simulink model "controlMCUSlugsMKII"  (Simulink 6.6)
settings: Solver=FixedStepDiscrete  StartTime=0.0  StopTime=10.0  FixedStep=0.01  RelTol=1e-3
InitFcn:
  | mcuInit
values from neighbouring files (symbols this model uses):
  apSampleTime = 0.01    [mcuInit.m]
  derivativesConstant = 5    [mcuInit.m]
  T = 0.01    [mcuInit.m]
undefined symbols (not defined in the file or in its folder): bankCommandLimit, baseHeight, bda, bde, bdr, bdt, bICda, bICde, bICdr, bICdt, controlMCUInit, daLimit, deLimit, drLimit, dtLimit, getAccBias, getAccels, getAttitude, getMidLevelCommands, getPassValues, getPidIdx, getVned, getWP, getXYZ, gsRead, ISA_g, lowRateTelemetryMavlink, mda, mde, mdr, mdt, mICda, mICde, mICdr, mICdt, pitchCommandLimit, protDecodeMavlink, readIpc, send2GS, setCurrentCommands, setDiagnosticFloat, setDiagnosticShort, setLogFloat1, setLogFloat2, setNavLat, setNavLong, setNavNav, u1, u2, updateEuler, updateLoad, updatePQR, updatePWM, updatePWM2, y1
libraries: dsPICdrivers x85, simulink x79, SLUGS_Library x23, aerolibconvert2 x5, aerolibutil x3
(part 4 of 5)

== system controlMCUSlugsMKII/Inner Loop/ Navigation/Lateral Channel/Bank to Psi Dot/Protect NaNs1 ==
  In1 : Inport
  Integer Delay3 : simulink/Discrete/Integer Delay  Orientation=left  vinit=0.0  samptime=T  NumDelays=1
  Relational Operator2 : RelationalOperator  Operator===  LogicOutDataTypeMode=Specify via dialog
  Switch3 : Switch  Criteria=u2 > Threshold  Threshold=0.3  SampleTime=.01
  Out1 : Outport  Orientation=down
  wires:
  Integer Delay3/1 -> Switch3/3
  Switch3/1 -> Out1/1, Integer Delay3/1
  In1/1 -> Relational Operator2/2, Relational Operator2/1, Switch3/1
  Relational Operator2/1 -> Switch3/2

== system controlMCUSlugsMKII/Inner Loop/ Navigation/Lateral Channel/Sideslip Compensation/Bank to Psi Dot ==
  phi_c : Inport
  U_m : Inport  Port=2
  Constant1 : Constant  Value=9.80665  OutDataTypeMode=single
  Divide : Product  Inputs=/*  OutDataTypeMode=single  OutScaling=2^-10  SampleTime=apSampleTime
  Divide1 : Product  OutDataTypeMode=single  OutScaling=2^-10  SampleTime=apSampleTime
  Subsystem8 : SLUGS_Library/Subsystem8  SystemSampleTime=-1
  bank Limit : Saturate  UpperLimit=bankCommandLimit  LowerLimit=-bankCommandLimit
  negprotect : Stateflow chart
  psi_dot_c : Outport
  wires:
  U_m/1 -> negprotect/1(val)
  Constant1/1 -> Divide/2
  Divide1/1 -> psi_dot_c/1
  Subsystem8/1 -> Divide1/1
  phi_c/1 -> bank Limit/1
  Divide/1 -> Divide1/2
  negprotect/1(zpVal) -> Divide/1
  bank Limit/1 -> Subsystem8/1

== system controlMCUSlugsMKII/Inner Loop/ Navigation/Lateral Channel/Sideslip Compensation/Low Pass ==
  a : Inport
  u : Inport  Port=2
  Compute Coef : Subsystem
  Detect Change : Subsystem
  Divide : Product  OutScaling=2^-10  SampleTime=apSampleTime
  Divide1 : Product  OutScaling=2^-10  SampleTime=apSampleTime
  IC : InitialCondition
  Integer Delay : simulink/Discrete/Integer Delay  vinit=0.0  samptime=apSampleTime  NumDelays=1
  Integer Delay1 : simulink/Discrete/Integer Delay  Orientation=left  vinit=0.0  samptime=apSampleTime  NumDelays=1
  Subtract : Sum  OutScaling=2^-10  SampleTime=apSampleTime
  y : Outport
  wires:
  Integer Delay1/1 -> Divide1/2
  u/1 -> Integer Delay/1
  IC/1 -> Compute Coef/Enable
  Subtract/1 -> Integer Delay1/1, y/1
  Divide1/1 -> Subtract/2
  Divide/1 -> Subtract/1
  Integer Delay/1 -> Divide/2
  Detect Change/1(change?) -> IC/1
  Compute Coef/2(c) -> Divide1/1
  Compute Coef/1(b) -> Divide/1
  a/1 -> Detect Change/1(Data), Compute Coef/1(a)

== system controlMCUSlugsMKII/Inner Loop/ Navigation/Lateral Channel/Sideslip Compensation/Protect NaNs2 ==
  In1 : Inport
  Integer Delay3 : simulink/Discrete/Integer Delay  Orientation=left  vinit=0.0  samptime=T  NumDelays=1
  Relational Operator2 : RelationalOperator  Operator===  LogicOutDataTypeMode=Specify via dialog
  Switch3 : Switch  Criteria=u2 > Threshold  Threshold=0.3  SampleTime=.01
  Out1 : Outport  Orientation=down
  wires:
  Relational Operator2/1 -> Switch3/2
  In1/1 -> Switch3/1, Relational Operator2/1, Relational Operator2/2
  Switch3/1 -> Integer Delay3/1, Out1/1
  Integer Delay3/1 -> Switch3/3

== system controlMCUSlugsMKII/Inner Loop/ Navigation/Lateral Channel/Sideslip Compensation/psi_dot to Bank ==
  psi_dot_c : Inport
  U_m : Inport  Port=2
  Constant1 : Constant  Value=9.80665  OutDataTypeMode=single
  Divide : Product  Inputs=**/  OutScaling=2^-10  SampleTime=apSampleTime
  Subsystem2 : SLUGS_Library/Subsystem2  SystemSampleTime=-1
  phi_c : Outport
  wires:
  psi_dot_c/1 -> Divide/1
  U_m/1 -> Divide/2
  Constant1/1 -> Divide/3
  Subsystem2/1 -> phi_c/1
  Divide/1 -> Subsystem2/1

== system controlMCUSlugsMKII/Inner Loop/ Navigation/Longitudinal Channel/Air Density from Height/Subsystem ==
  u : Inport
  v : Inport  Port=2
  C Function Call : dsPICdrivers/OTHERS/C Function Call  Tag=dsPIC_dsPIC_CFunctionCall  fctName='myPow'  INPUT_SIZE=1  INPUT1=real32  INPUT2=real32  INPUT3=--  OUTPUT_SIZE=1  OUTPUT1=real32  SampleTime=-1  InputType=[ 7 7 ]  OutputType=[ 7 ]  FctDeclaration=extern real32_T myPow(real32_T u1, real32_T u2);  FctCall=%y1 = myPow(%u1, %u2);  OrderingInOutPopup=None
  u^v : Outport
  wires:
  v/1 -> C Function Call/2
  u/1 -> C Function Call/1
  C Function Call/1 -> u^v/1

== system controlMCUSlugsMKII/Inner Loop/ Navigation/Longitudinal Channel/Airspeed Hold [PID]/Trapezoidal Integrator ==
  x : Inport
  Reset : Inport  Port=2
  Constant : Constant  Value=1/3  OutDataTypeMode=single
  Constant1 : Constant  Value=4/3  OutDataTypeMode=single
  Constant2 : Constant  Value=T/2  OutDataTypeMode=single
  Constant3 : Constant  Value=1/3  OutDataTypeMode=single
  Constant5 : Constant  Orientation=left  Value=0  OutDataTypeMode=single
  Integer Delay : simulink/Discrete/Integer Delay  vinit=0.0  samptime=T  NumDelays=1
  Integer Delay1 : simulink/Discrete/Integer Delay  vinit=0.0  samptime=T  NumDelays=2
  Integer Delay2 : simulink/Discrete/Integer Delay  Orientation=left  vinit=0.0  samptime=T  NumDelays=1
  Product{,1..3} (4 alike) : Product  OutDataTypeMode=single  RndMeth=Zero
  "Protect NaNs " : Subsystem
  Protect NaNs1 : Subsystem
  Subtract : Sum  Inputs=3  OutDataTypeMode=single  OutScaling=2^-10
  Subtract1 : Sum  Inputs=2  OutDataTypeMode=single  OutScaling=2^-10
  Switch1 : Switch  Criteria=u2 > Threshold  Threshold=0.3  SampleTime=.01
  Int(x) : Outport
  wires:
  "Protect NaNs "/1(Out1) -> Product/1, Integer Delay/1, Integer Delay1/1
  Protect NaNs1/1(Out1) -> Int(x)/1, Integer Delay2/1
  Constant/1 -> Product/2
  Constant1/1 -> Product1/2
  Integer Delay/1 -> Product1/1
  Integer Delay1/1 -> Product2/1
  Constant3/1 -> Product2/2
  x/1 -> "Protect NaNs "/1(In1)
  Product/1 -> Subtract/1
  Product1/1 -> Subtract/2
  Product2/1 -> Subtract/3
  Constant2/1 -> Product3/1
  Subtract/1 -> Product3/2
  Subtract1/1 -> Switch1/3
  Integer Delay2/1 -> Subtract1/1
  Product3/1 -> Subtract1/2
  Constant5/1 -> Switch1/1
  Reset/1 -> Switch1/2
  Switch1/1 -> Protect NaNs1/1(In1)

== system controlMCUSlugsMKII/Inner Loop/ Navigation/Longitudinal Channel/Compute Airspeed/Subsystem1 ==
  x : Inport
  C Function Call : dsPICdrivers/OTHERS/C Function Call  Tag=dsPIC_dsPIC_CFunctionCall  fctName='mySqrt'  INPUT_SIZE=1  INPUT1=real32  INPUT2=--  INPUT3=--  OUTPUT_SIZE=1  OUTPUT1=real32  SampleTime=-1  InputType=[ 7 ]  OutputType=[ 7 ]  FctDeclaration=extern real32_T mySqrt(real32_T u1);  FctCall=%y1 = mySqrt(%u1);  OrderingInOutPopup=None
  negprotect : Stateflow chart
  sqrt(x) : Outport
  wires:
  x/1 -> negprotect/1(val)
  negprotect/1(zpVal) -> C Function Call/1
  C Function Call/1 -> sqrt(x)/1

== system controlMCUSlugsMKII/Inner Loop/ Navigation/Navigation/Compute Lateral Error/Subsystem3 ==
  x : Inport
  y : Inport  Port=2
  Dot Product : simulink/Math Operations/Dot Product  InputSameDT=on  OutDataType=sfix(16)  OutScaling=2^-10  DoSatur=off
  Embedded MATLAB Function : Stateflow chart
  Environment Controller : simulink/Signal Routing/Environment Controller  SystemSampleTime=-1
  Protect NaNs : Subsystem
  x dot y : Outport
  wires:
  Environment Controller/1 -> Protect NaNs/1(In1)
  Embedded MATLAB Function/1(xDoty) -> Environment Controller/2
  Dot Product/1 -> Environment Controller/1
  x/1 -> Dot Product/1, Embedded MATLAB Function/1(x)
  y/1 -> Dot Product/2, Embedded MATLAB Function/2(y)
  Protect NaNs/1(Out1) -> x dot y/1

== system controlMCUSlugsMKII/Inner Loop/ Navigation/Navigation/Compute WP Index/Compute P ==
  WP1 : Inport  Orientation=left
  T1 : Inport  Port=2
  WP2 : Inport  Orientation=left  Port=3
  U_com : Inport  Port=4
  GS R_in : Inport  Orientation=left  Port=5
  GS LLA : Inport  Orientation=left  Port=6
  Groundspeed : Inport  Port=7
  Preturn Constant : Inport  Port=8
  Enable : EnablePort
  Add : Sum  Inputs=2  OutScaling=2^-10
  Compute R : Subsystem
  Compute T  in Frenet : Subsystem  Orientation=left  AncestorBlock=SLUGS_Library/Navigation/Compute Frenet
  Demux : Demux  Orientation=left  Outputs=3
  Geod2LTP1 : Subsystem  Orientation=left
      mask Description:
      | This block provides transformation of the Geodetic coordinates
      | to the LTP coorinate system. The block uses two consecutive transformations
      | (Geodetic -> ECEF ->LTP).
      | Geodetic coordinates of the LTP origin should also be predetermined.
      mask Help: Oops!
      mask Display: plot(0,0,100,100,[45,40,35,40,40],[85,95,85,95,40],[85,95,85,95,40],[35,40,45,40,40],[60,40,10,20,10,14],[70,40,10,13,10,20],[56,45],[70,70],[60,60],[50,60],[60,60],[30,40],[50,60],[20,20],[30,40],[20,20],[45,55],[35,25],[75,65],[35,25])
  Get Circles : Subsystem
  IC : InitialCondition  Value=50
  Integer Delay1 : simulink/Discrete/Integer Delay  vinit=0.0  samptime=-1  NumDelays=1
  Integer Delay2 : simulink/Discrete/Integer Delay  Orientation=left  vinit=0.0  samptime=-1  NumDelays=1
  Product1 : Product  OutDataTypeMode=single  RndMeth=Zero
  WP1_1 : InportShadow  Port=1  LatchByCopyingInsideSignal=off
  get WP Coord from Index : Subsystem  Orientation=left  AncestorBlock=SLUGS_Library/Navigation/get WP Coord from Index
  P : Outport  InitialOutput=50
  wires:
  IC/1 -> P/1
  GS LLA/1 -> Geod2LTP1/1(GS Lat,Lon)
  GS R_in/1 -> Geod2LTP1/2(GS ECEF)
  get WP Coord from Index/1(WP Coord) -> Demux/1
  Geod2LTP1/1("NEU, m") -> Integer Delay2/1
  Demux/3 -> Geod2LTP1/5(Hight,m(GPS))
  Demux/2 -> Geod2LTP1/4("Lon, deg(GPS)")
  Demux/1 -> Geod2LTP1/3("Lat, deg(GPS)")
  Integer Delay1/1 -> Get Circles/1(T1)
  WP1_1/1 -> Get Circles/3("Wp_to ")
  T1/1 -> Integer Delay1/1
  WP2/1 -> get WP Coord from Index/1(WP Idx)
  WP1/1 -> Compute T  in Frenet/1(Pos 1)
  Compute T  in Frenet/1(T) -> Get Circles/2(T2)
  Integer Delay2/1 -> Compute T  in Frenet/2(Pos 2)
  Compute R/1(R) -> Get Circles/4(R)
  U_com/1 -> Compute R/1(U_com)
  Product1/1 -> Add/1
  Groundspeed/1 -> Product1/2
  Preturn Constant/1 -> Product1/1
  Get Circles/1(P) -> Add/2
  Add/1 -> IC/1

== system controlMCUSlugsMKII/Inner Loop/ Navigation/Navigation/Compute WP Index/Grab IC ==
  UAV Pos : Inport
  Enable : EnablePort
  Compute GS Location : Subsystem
  Constant : Constant  Value=11  OutDataTypeMode=uint8
  Selector : Selector  IndexOptions=Index vector (dialog)  Indices=[3 1 2]  OutputSizes=1  InputPortWidth=3
  get GS Location (WP 11 is GS) : Subsystem  AncestorBlock=SLUGS_Library/Navigation/get WP Coord from Index
  IC : Outport
  "GS, Lat Lon" : Outport  Port=2
  GS R_in : Outport  Port=3
  wires:
  get GS Location (WP 11 is GS)/1(WP Coord) -> Selector/1
  Selector/1 -> Compute GS Location/1(GS Location)
  Compute GS Location/2(R_in) -> GS R_in/1
  Compute GS Location/1("Lat, Lon") -> "GS, Lat Lon"/1
  Constant/1 -> get GS Location (WP 11 is GS)/1(WP Idx)
  UAV Pos/1 -> IC/1

== system controlMCUSlugsMKII/Inner Loop/ Navigation/Navigation/Compute WP Index/Protect NaNs ==
  In1 : Inport
  Integer Delay3 : simulink/Discrete/Integer Delay  Orientation=left  vinit=0.0  samptime=T  NumDelays=1
  Relational Operator2 : RelationalOperator  Operator===  LogicOutDataTypeMode=Specify via dialog
  Switch3 : Switch  Criteria=u2 > Threshold  Threshold=0.3  SampleTime=.01
  Out1 : Outport  Orientation=down
  wires:
  Relational Operator2/1 -> Switch3/2
  In1/1 -> Switch3/1, Relational Operator2/1, Relational Operator2/2
  Switch3/1 -> Integer Delay3/1, Out1/1
  Integer Delay3/1 -> Switch3/3

== system controlMCUSlugsMKII/Inner Loop/ Navigation/Navigation/Compute WP Index/Subsystem ==
  WP Fly : Inport
  Add1 : Sum  Inputs=2  OutScaling=2^-10
  Hit  Crossing1 : HitCross  HitCrossingOffset=0.3  HitCrossingDirection=rising  SampleTime=apSampleTime
  Integer Delay1 : simulink/Discrete/Integer Delay  vinit=0  samptime=-1  NumDelays=1
  Just Enab : Outport
  wires:
  WP Fly/1 -> Hit  Crossing1/1
  Add1/1 -> Just Enab/1
  Hit  Crossing1/1 -> Integer Delay1/1, Add1/2
  Integer Delay1/1 -> Add1/1

== system controlMCUSlugsMKII/Inner Loop/ Navigation/Navigation/Compute WP Index/Subsystem1 ==
  swInc : Inport  Orientation=down
  Add : Sum  Orientation=left  Inputs=2  OutScaling=2^-10
  IC : InitialCondition  Orientation=down
  Integer Delay2 : simulink/Discrete/Integer Delay  Orientation=left  vinit=0  samptime=-1  NumDelays=1
  swEna : Outport  Orientation=left
  wires:
  swInc/1 -> IC/1
  Add/1 -> swEna/1
  IC/1 -> Add/2, Integer Delay2/1
  Integer Delay2/1 -> Add/1

== system controlMCUSlugsMKII/Inner Loop/ Navigation/Navigation/Compute WP Index/Switch when  in Line Segment ==
  P : Inport
  WP0 Idx : Inport  Port=2
  Puav : Inport  Port=3
  "WP1 " : Inport  Port=4
  WP0 : Inport  Port=5
  T : Inport  Port=6
  1st WP : Switch  Criteria=u2 > Threshold  Threshold=0.3
  Compare To Zero : simulink/Logic and Bit Operations/Compare To Zero  SystemSampleTime=-1  relop=>  LogicOutDataTypeMode=uint8  ZeroCross=off
  Compute  Projection : Subsystem
  Compute Total Run : Subsystem
  IC : InitialCondition
  Integer Delay1 : simulink/Discrete/Integer Delay  vinit=0  samptime=-1  NumDelays=1
  Subsystem1 : Subsystem
  Switch Distance Less than? : RelationalOperator  LogicOutDataTypeMode=Specify via dialog  SampleTime=apSampleTime
  Switch Distance WP0 : Constant  Value=100  OutDataTypeMode=single
  WP Update : Subsystem  mask{T=0.01}
      mask prompts: T "Sample Time"
  "WP0   " : InportShadow  Port=5  LatchByCopyingInsideSignal=off
  Switch LS : Outport
  Tot Run : Outport  Port=2
  Dg : Outport  Port=3
  wires:
  Compute  Projection/1(Dg) -> Switch Distance Less than?/1, Dg/1
  Subsystem1/1(swEna) -> IC/1
  WP Update/1(Update?) -> Subsystem1/1(swInc)
  "WP0   "/1 -> WP Update/1(XYZ), Compute Total Run/2("WP0  ")
  "WP1 "/1 -> Compute Total Run/1(WP1)
  Compute Total Run/1(Tot Run) -> Switch Distance Less than?/2, Tot Run/1
  Puav/1 -> Compute  Projection/1(Puav)
  WP0/1 -> Compute  Projection/2(WP0)
  T/1 -> Compute  Projection/3(T)
  Switch Distance Less than?/1 -> Switch LS/1
  WP0 Idx/1 -> Integer Delay1/1
  P/1 -> 1st WP/1
  1st WP/1 -> Compute Total Run/3(P)
  Integer Delay1/1 -> Compare To Zero/1
  Switch Distance WP0/1 -> 1st WP/3
  Compare To Zero/1 -> 1st WP/2
  IC/1 -> Compute Total Run/Enable

== system controlMCUSlugsMKII/Inner Loop/ Navigation/Navigation/Get Wps Compute Frenet/Geod2LTP1 ==
  GS Lat,Lon : Inport
  GS ECEF : Inport  Port=2
  "Lat, deg(GPS)" : Inport  Port=3
  "Lon, deg(GPS)" : Inport  Port=4
  Hight,m(GPS) : Inport  Port=5
  ECEF2LTP (UEN) : Subsystem
      mask Display: plot(0,0,100,100,[45,40,35,40,40],[85,95,85,95,40],[85,95,85,95,40],[35,40,45,40,40],[60,40,10,20,10,14],[70,40,10,13,10,20],[56,45],[70,70],[60,60],[50,60],[60,60],[30,40],[50,60],[20,20],[30,40],[20,20],[45,55],[35,25],[75,65],[35,25])
  Geod2ECEF1 : Subsystem  mask{Re=6378137, Rp=6356752.3142}
      mask prompts: Re "Enter equatorial radius, m"; Rp "Enter polar radius,m"
  Mux : Mux  Inputs=3
  Reshape : Reshape  OutputDimensionality=Column vector (2-D)
  Reshape1 : Reshape
  Sum1 : Sum  Inputs=|+-  OutDataTypeMode=single  SaturateOnIntegerOverflow=on
  UEN 2 NEU : Gain  Gain=[0 0 1;0 1 0;1 0 0]  Multiplication=Matrix(K*u)  OutDataTypeMode=Specify via dialog  OutDataType=float('single')  SaturateOnIntegerOverflow=on
  "NEU, m" : Outport
  wires:
  UEN 2 NEU/1 -> Reshape1/1
  Geod2ECEF1/3("Ze, m ") -> Mux/3
  Geod2ECEF1/1("Xe, m ") -> Mux/1
  Geod2ECEF1/2("Ye, m ") -> Mux/2
  "Lat, deg(GPS)"/1 -> Geod2ECEF1/2("lat, deg")
  "Lon, deg(GPS)"/1 -> Geod2ECEF1/3(lon,deg)
  GS Lat,Lon/1 -> ECEF2LTP (UEN)/2("Long, Lat")
  GS ECEF/1 -> Sum1/2
  ECEF2LTP (UEN)/1(Out) -> Reshape/1  "Moving Side"
  Hight,m(GPS)/1 -> Geod2ECEF1/1("height, m")
  Mux/1 -> Sum1/1  "r_mov"
  Sum1/1 -> ECEF2LTP (UEN)/1(ECEF coordinates)
  Reshape/1 -> UEN 2 NEU/1
  Reshape1/1 -> "NEU, m"/1

== system controlMCUSlugsMKII/Inner Loop/ Navigation/Navigation/Get Wps Compute Frenet/Geod2LTP2 ==
  GS Lat,Lon : Inport
  GS ECEF : Inport  Port=2
  "Lat, deg(GPS)" : Inport  Port=3
  "Lon, deg(GPS)" : Inport  Port=4
  Hight,m(GPS) : Inport  Port=5
  ECEF2LTP (UEN) : Subsystem
      mask Display: plot(0,0,100,100,[45,40,35,40,40],[85,95,85,95,40],[85,95,85,95,40],[35,40,45,40,40],[60,40,10,20,10,14],[70,40,10,13,10,20],[56,45],[70,70],[60,60],[50,60],[60,60],[30,40],[50,60],[20,20],[30,40],[20,20],[45,55],[35,25],[75,65],[35,25])
  Geod2ECEF1 : Subsystem  mask{Re=6378137, Rp=6356752.3142}
      mask prompts: Re "Enter equatorial radius, m"; Rp "Enter polar radius,m"
  Mux : Mux  Inputs=3
  Reshape : Reshape  OutputDimensionality=Column vector (2-D)
  Reshape1 : Reshape
  Sum1 : Sum  Inputs=|+-  OutDataTypeMode=single  SaturateOnIntegerOverflow=on
  UEN 2 NEU : Gain  Gain=[0 0 1;0 1 0;1 0 0]  Multiplication=Matrix(K*u)  OutDataTypeMode=Specify via dialog  OutDataType=float('single')  SaturateOnIntegerOverflow=on
  "NEU, m" : Outport
  wires:
  UEN 2 NEU/1 -> Reshape1/1
  Geod2ECEF1/3("Ze, m ") -> Mux/3
  Geod2ECEF1/1("Xe, m ") -> Mux/1
  Geod2ECEF1/2("Ye, m ") -> Mux/2
  "Lat, deg(GPS)"/1 -> Geod2ECEF1/2("lat, deg")
  "Lon, deg(GPS)"/1 -> Geod2ECEF1/3(lon,deg)
  GS Lat,Lon/1 -> ECEF2LTP (UEN)/2("Long, Lat")
  GS ECEF/1 -> Sum1/2
  ECEF2LTP (UEN)/1(Out) -> Reshape/1  "Moving Side"
  Hight,m(GPS)/1 -> Geod2ECEF1/1("height, m")
  Mux/1 -> Sum1/1  "r_mov"
  Sum1/1 -> ECEF2LTP (UEN)/1(ECEF coordinates)
  Reshape/1 -> UEN 2 NEU/1
  Reshape1/1 -> "NEU, m"/1

== system controlMCUSlugsMKII/Inner Loop/ Navigation/Navigation/Get Wps Compute Frenet/get WP Coord from Index ==
  WP Idx : Inport
  C Function Call : dsPICdrivers/OTHERS/C Function Call  Tag=dsPIC_dsPIC_CFunctionCall  fctName='getWP'  INPUT_SIZE=1  INPUT1=uint8  INPUT2=--  INPUT3=--  OUTPUT_SIZE=3  OUTPUT1=real32  SampleTime=-1  InputType=[ 2 ]  OutputType=[ 7 ]  FctDeclaration=extern void getWP(uint8_T u1,real32_T* y1);  FctCall=getWP(%u1, *%y1);  OrderingInOutPopup=None
  WP Coord : Outport
  wires:
  WP Idx/1 -> C Function Call/1
  C Function Call/1 -> WP Coord/1

== system controlMCUSlugsMKII/Inner Loop/ Navigation/Navigation/Get Wps Compute Frenet/get WP Coord from Index  ==
  WP Idx : Inport
  C Function Call : dsPICdrivers/OTHERS/C Function Call  Tag=dsPIC_dsPIC_CFunctionCall  fctName='getWP'  INPUT_SIZE=1  INPUT1=uint8  INPUT2=--  INPUT3=--  OUTPUT_SIZE=3  OUTPUT1=real32  SampleTime=-1  InputType=[ 2 ]  OutputType=[ 7 ]  FctDeclaration=extern void getWP(uint8_T u1,real32_T* y1);  FctCall=getWP(%u1, *%y1);  OrderingInOutPopup=None
  WP Coord : Outport
  wires:
  WP Idx/1 -> C Function Call/1
  C Function Call/1 -> WP Coord/1

== system controlMCUSlugsMKII/Inner Loop/ Navigation/Navigation/Park, Deyst & How Lat Accel Cmd/Compute Eta ==
  Vxyz : Inport
  L2_vec : Inport  Port=2
  Ground Speed : Inport  Port=3
  3x3 Cross Product : aerolibutil/3x3 Cross Product  SystemSampleTime=-1
  Divide5 : Product  Inputs=*//  OutScaling=2^-10
  Norm : SLUGS_Library/Navigation/Norm  SystemSampleTime=-1
  Selector : Selector  IndexOptions=Index vector (dialog)  Indices=[3]  OutputSizes=1  InputPortWidth=3
  Subsystem6 : Subsystem  AncestorBlock=SLUGS_Library/Subsystem6
  To Workspace : ToWorkspace  VariableName=L1  SampleTime=-1  SaveFormat=Array
  To Workspace1 : ToWorkspace  VariableName=Vned  SampleTime=-1  SaveFormat=Array
  To Workspace2 : ToWorkspace  VariableName=eta  SampleTime=-1  SaveFormat=Array
  "[-25 25]" : Saturate  UpperLimit=25  LowerLimit=-25  SampleTime=.01
  negprotect : Stateflow chart
  Eta : Outport
  wires:
  negprotect/1(zpVal) -> Divide5/2
  L2_vec/1 -> To Workspace/1, 3x3 Cross Product/2, Norm/1
  Divide5/1 -> Selector/1
  Norm/1 -> negprotect/1(val)
  3x3 Cross Product/1 -> Divide5/1
  Vxyz/1 -> "[-25 25]"/1
  Selector/1 -> Subsystem6/1(x)
  Subsystem6/1(asin(x)) -> Eta/1, To Workspace2/1
  Ground Speed/1 -> Divide5/3
  "[-25 25]"/1 -> 3x3 Cross Product/1, To Workspace1/1

== system controlMCUSlugsMKII/Inner Loop/ Navigation/Navigation/Park, Deyst & How Lat Accel Cmd/Compute L2 Vector LINE MODE ==
  Pe_lat : Inport
  L2 : Inport  Port=2
  T : Inport  Port=3
  N : Inport  Port=4
  Add : Sum  Inputs=-+  OutScaling=2^-10
  Add2 : Sum  Inputs=-+  OutScaling=2^-10
  Divide{,1..3} (4 alike) : Product  OutScaling=2^-10
  Gain : Gain  Orientation=up  Gain=-1
  Subsystem1 : SLUGS_Library/Subsystem1  SystemSampleTime=-1
  Subsystem9 : SLUGS_Library/Subsystem9  SystemSampleTime=-1
  To Workspace3 : ToWorkspace  VariableName=Pey  SampleTime=-1  SaveFormat=Array
  L2_vec : Outport
  wires:
  Divide3/1 -> Add2/2  "||CD||*T"
  T/1 -> Divide3/1
  N/1 -> Divide2/1
  Divide2/1 -> Add2/1  "N*Pey"
  Subsystem1/1 -> Divide3/2  "||CD||"
  Add/1 -> Subsystem9/1
  Divide/1 -> Add/2
  Divide1/1 -> Add/1
  Pe_lat/1 -> Divide1/1, Divide1/2, To Workspace3/1, Gain/1
  L2/1 -> Divide/2, Divide/1
  Gain/1 -> Divide2/2
  Add2/1 -> L2_vec/1  "L1_vec"
  Subsystem9/1 -> Subsystem1/1

== system controlMCUSlugsMKII/Inner Loop/ Navigation/Navigation/Park, Deyst & How Lat Accel Cmd/GainSchedule L2 and Get Groundspeed ==
  L2 Base : Inport
  Vxyz : Inport  Port=2
  Divide4 : Product  OutScaling=2^-10
  "Norm " : Subsystem  AncestorBlock=SLUGS_Library/Navigation/Norm
  Protect NaNs : Subsystem
  To Workspace3 : ToWorkspace  VariableName=L2  SampleTime=-1  SaveFormat=Array
  "[0 45]" : Saturate  UpperLimit=45  LowerLimit=0  SampleTime=.01
  negprotect1 : Stateflow chart
  L2 : Outport
  Ground Speed : Outport  Port=2
  wires:
  Divide4/1 -> To Workspace3/1, L2/1
  L2 Base/1 -> Divide4/1
  negprotect1/1(zpVal) -> Protect NaNs/1(In1)
  Vxyz/1 -> "Norm "/1(Vector)
  "Norm "/1(Norm) -> negprotect1/1(val)
  Protect NaNs/1(Out1) -> "[0 45]"/1
  "[0 45]"/1 -> Divide4/2, Ground Speed/1

== system controlMCUSlugsMKII/Inner Loop/ Navigation/Navigation/Park, Deyst & How Lat Accel Cmd/Park's Lateral Accel Command ==
  L2 : Inport
  eta : Inport  Port=2
  Ground Speed : Inport  Port=3
  Constant : Constant  Value=2
  Product : Product  Inputs=***/*  RndMeth=Zero
  Protect NaNs : Subsystem
  Subsystem7 : SLUGS_Library/Subsystem7  SystemSampleTime=-1
  "[-25,25]" : Saturate  UpperLimit=25  LowerLimit=-25
  a_s_c : Outport
  wires:
  Product/1 -> Protect NaNs/1(In1)
  Subsystem7/1 -> Product/5
  L2/1 -> Product/4
  Constant/1 -> Product/3
  Ground Speed/1 -> Product/2, Product/1
  eta/1 -> Subsystem7/1
  Protect NaNs/1(Out1) -> "[-25,25]"/1
  "[-25,25]"/1 -> a_s_c/1

== system controlMCUSlugsMKII/Inner Loop/ Navigation/Navigation/as_c to phi_c/Protect NaNs ==
  In1 : Inport
  Integer Delay3 : simulink/Discrete/Integer Delay  Orientation=left  vinit=0.0  samptime=T  NumDelays=1
  Relational Operator2 : RelationalOperator  Operator===  LogicOutDataTypeMode=Specify via dialog
  Switch3 : Switch  Criteria=u2 > Threshold  Threshold=0.3  SampleTime=.01
  Out1 : Outport  Orientation=down
  wires:
  Relational Operator2/1 -> Switch3/2
  In1/1 -> Switch3/1, Relational Operator2/1, Relational Operator2/2
  Switch3/1 -> Integer Delay3/1, Out1/1
  Integer Delay3/1 -> Switch3/3

== system controlMCUSlugsMKII/Update PWM Commands and Send Telemetry/Generate PWM Signals Based on the Control Type/If  Control Type Is Selective Passthrough/Convert to PWM ==
  " Angle(rad)" : Inport  Orientation=down
  Add : Sum  OutScaling=2^-10
  Constant1 : Constant  Value=slopem
  Constant2 : Constant  Value=interceptb
  Data Type Conversion : DataTypeConversion  OutDataTypeMode=uint16
  Divide : Product  OutScaling=2^-10
  PWM : Outport
  wires:
  Data Type Conversion/1 -> PWM/1
  " Angle(rad)"/1 -> Divide/1
  Constant2/1 -> Add/2
  Divide/1 -> Add/1
  Add/1 -> Data Type Conversion/1
  Constant1/1 -> Divide/2

== system controlMCUSlugsMKII/Update PWM Commands and Send Telemetry/Generate PWM Signals Based on the Control Type/If  Control Type Is Selective Passthrough/Convert to PWM1 ==
  " Angle(rad)" : Inport  Orientation=down
  Add : Sum  OutScaling=2^-10
  Constant1 : Constant  Value=slopem
  Constant2 : Constant  Value=interceptb
  Data Type Conversion : DataTypeConversion  OutDataTypeMode=uint16
  Divide : Product  OutScaling=2^-10
  PWM : Outport
  wires:
  Constant1/1 -> Divide/2
  Add/1 -> Data Type Conversion/1
  Divide/1 -> Add/1
  Constant2/1 -> Add/2
  " Angle(rad)"/1 -> Divide/1
  Data Type Conversion/1 -> PWM/1

== system controlMCUSlugsMKII/Update PWM Commands and Send Telemetry/Generate PWM Signals Based on the Control Type/If  Control Type Is Selective Passthrough/Convert to PWM2 ==
  " Angle(rad)" : Inport  Orientation=down
  Add : Sum  OutScaling=2^-10
  Constant1 : Constant  Value=slopem
  Constant2 : Constant  Value=interceptb
  Data Type Conversion : DataTypeConversion  OutDataTypeMode=uint16
  Divide : Product  OutScaling=2^-10
  PWM : Outport
  wires:
  Data Type Conversion/1 -> PWM/1
  " Angle(rad)"/1 -> Divide/1
  Constant2/1 -> Add/2
  Divide/1 -> Add/1
  Add/1 -> Data Type Conversion/1
  Constant1/1 -> Divide/2

== system controlMCUSlugsMKII/Update PWM Commands and Send Telemetry/Generate PWM Signals Based on the Control Type/If  Control Type Is Selective Passthrough/Convert to PWM3 ==
  " Angle(rad)" : Inport  Orientation=down
  Add : Sum  OutScaling=2^-10
  Constant1 : Constant  Value=slopem
  Constant2 : Constant  Value=interceptb
  Data Type Conversion : DataTypeConversion  OutDataTypeMode=uint16
  Divide : Product  OutScaling=2^-10
  PWM : Outport
  wires:
  Constant1/1 -> Divide/2
  Add/1 -> Data Type Conversion/1
  Divide/1 -> Add/1
  Constant2/1 -> Add/2
  " Angle(rad)"/1 -> Divide/1
  Data Type Conversion/1 -> PWM/1

== system controlMCUSlugsMKII/Update PWM Commands and Send Telemetry/Generate PWM Signals Based on the Control Type/If  Control Type Is Wp Follow  or Inner Cmds/Convert to PWM ==
  " Angle(rad)" : Inport  Orientation=down
  Add : Sum  OutScaling=2^-10
  Constant1 : Constant  Value=slopem
  Constant2 : Constant  Value=interceptb
  Data Type Conversion : DataTypeConversion  OutDataTypeMode=uint16
  Divide : Product  OutScaling=2^-10
  PWM : Outport
  wires:
  Data Type Conversion/1 -> PWM/1
  " Angle(rad)"/1 -> Divide/1
  Constant2/1 -> Add/2
  Divide/1 -> Add/1
  Add/1 -> Data Type Conversion/1
  Constant1/1 -> Divide/2

== system controlMCUSlugsMKII/Update PWM Commands and Send Telemetry/Generate PWM Signals Based on the Control Type/If  Control Type Is Wp Follow  or Inner Cmds/Convert to PWM1 ==
  " Angle(rad)" : Inport  Orientation=down
  Add : Sum  OutScaling=2^-10
  Constant1 : Constant  Value=slopem
  Constant2 : Constant  Value=interceptb
  Data Type Conversion : DataTypeConversion  OutDataTypeMode=uint16
  Divide : Product  OutScaling=2^-10
  PWM : Outport
  wires:
  Constant1/1 -> Divide/2
  Add/1 -> Data Type Conversion/1
  Divide/1 -> Add/1
  Constant2/1 -> Add/2
  " Angle(rad)"/1 -> Divide/1
  Data Type Conversion/1 -> PWM/1

== system controlMCUSlugsMKII/Update PWM Commands and Send Telemetry/Generate PWM Signals Based on the Control Type/If  Control Type Is Wp Follow  or Inner Cmds/Convert to PWM2 ==
  " Angle(rad)" : Inport  Orientation=down
  Add : Sum  OutScaling=2^-10
  Constant1 : Constant  Value=slopem
  Constant2 : Constant  Value=interceptb
  Data Type Conversion : DataTypeConversion  OutDataTypeMode=uint16
  Divide : Product  OutScaling=2^-10
  PWM : Outport
  wires:
  Data Type Conversion/1 -> PWM/1
  " Angle(rad)"/1 -> Divide/1
  Constant2/1 -> Add/2
  Divide/1 -> Add/1
  Add/1 -> Data Type Conversion/1
  Constant1/1 -> Divide/2

== system controlMCUSlugsMKII/Update PWM Commands and Send Telemetry/Generate PWM Signals Based on the Control Type/If  Control Type Is Wp Follow  or Inner Cmds/Convert to PWM3 ==
  " Angle(rad)" : Inport  Orientation=down
  Add : Sum  OutScaling=2^-10
  Constant1 : Constant  Value=slopem
  Constant2 : Constant  Value=interceptb
  Data Type Conversion : DataTypeConversion  OutDataTypeMode=uint16
  Divide : Product  OutScaling=2^-10
  PWM : Outport
  wires:
  Constant1/1 -> Divide/2
  Add/1 -> Data Type Conversion/1
  Divide/1 -> Add/1
  Constant2/1 -> Add/2
  " Angle(rad)"/1 -> Divide/1
  Data Type Conversion/1 -> PWM/1

== system controlMCUSlugsMKII/Inner Loop/ Navigation/L1 Output Feedback Controller With  Projection Operator/Control  Law/Compute Coef/Subsystem11 ==
  u : Inport
  C Function Call : dsPICdrivers/OTHERS/C Function Call  Tag=dsPIC_dsPIC_CFunctionCall  fctName='myExp'  INPUT_SIZE=1  INPUT1=real32  INPUT2=--  INPUT3=--  OUTPUT_SIZE=1  OUTPUT1=real32  SampleTime=-1  InputType=[ 7 ]  OutputType=[ 7 ]  FctDeclaration=extern real32_T myExp(real32_T u1);  FctCall=%y1 = myExp(%u1);  OrderingInOutPopup=None
  exp(u) : Outport
  wires:
  C Function Call/1 -> exp(u)/1
  u/1 -> C Function Call/1

== system controlMCUSlugsMKII/Inner Loop/ Navigation/L1 Output Feedback Controller With  Projection Operator/State Predictor/Compute Coef/Subsystem11 ==
  u : Inport
  C Function Call : dsPICdrivers/OTHERS/C Function Call  Tag=dsPIC_dsPIC_CFunctionCall  fctName='myExp'  INPUT_SIZE=1  INPUT1=real32  INPUT2=--  INPUT3=--  OUTPUT_SIZE=1  OUTPUT1=real32  SampleTime=-1  InputType=[ 7 ]  OutputType=[ 7 ]  FctDeclaration=extern real32_T myExp(real32_T u1);  FctCall=%y1 = myExp(%u1);  OrderingInOutPopup=None
  exp(u) : Outport
  wires:
  u/1 -> C Function Call/1
  C Function Call/1 -> exp(u)/1

== system controlMCUSlugsMKII/Inner Loop/ Navigation/Lateral Channel/Sideslip Compensation/Low Pass/Compute Coef ==
  a : Inport
  Enable : EnablePort
  -T : Gain  Gain=-apSampleTime  SampleTime=apSampleTime
  1-c : Sum  Inputs=-+  OutDataTypeMode=single  OutScaling=2^-10  SampleTime=apSampleTime
  Constant : Constant
  Math Function : Math  SaturateOnIntegerOverflow=on
  b : Outport
  c : Outport  Port=2
  wires:
  a/1 -> -T/1
  1-c/1 -> b/1
  Constant/1 -> 1-c/2
  Math Function/1 -> c/1, 1-c/1  "c"
  -T/1 -> Math Function/1

== system controlMCUSlugsMKII/Inner Loop/ Navigation/Lateral Channel/Sideslip Compensation/Low Pass/Detect Change ==
  Data : Inport
  Abs1 : Abs  SampleTime=apSampleTime
  Difference1 : simulink/Discrete/Difference  SystemSampleTime=-1  ICPrevInput=0.0  OutDataType=sfix(16)  OutScaling=2^-10  DoSatur=off
  Saturation1 : Saturate  UpperLimit=1  LowerLimit=0  SampleTime=apSampleTime
  change? : Outport
  wires:
  Saturation1/1 -> change?/1
  Data/1 -> Difference1/1
  Abs1/1 -> Saturation1/1
  Difference1/1 -> Abs1/1

== system controlMCUSlugsMKII/Inner Loop/ Navigation/Longitudinal Channel/Airspeed Hold [PID]/Trapezoidal Integrator/Protect NaNs  ==
  In1 : Inport
  Integer Delay3 : simulink/Discrete/Integer Delay  Orientation=left  vinit=0.0  samptime=T  NumDelays=1
  Relational Operator2 : RelationalOperator  Operator===  LogicOutDataTypeMode=Specify via dialog
  Switch3 : Switch  Criteria=u2 > Threshold  Threshold=0.3  SampleTime=.01
  Out1 : Outport  Orientation=down
  wires:
  Relational Operator2/1 -> Switch3/2
  In1/1 -> Switch3/1, Relational Operator2/1, Relational Operator2/2
  Switch3/1 -> Integer Delay3/1, Out1/1
  Integer Delay3/1 -> Switch3/3

== system controlMCUSlugsMKII/Inner Loop/ Navigation/Longitudinal Channel/Airspeed Hold [PID]/Trapezoidal Integrator/Protect NaNs1 ==
  In1 : Inport
  Integer Delay3 : simulink/Discrete/Integer Delay  Orientation=left  vinit=0.0  samptime=T  NumDelays=1
  Relational Operator2 : RelationalOperator  Operator===  LogicOutDataTypeMode=Specify via dialog
  Switch3 : Switch  Criteria=u2 > Threshold  Threshold=0.3  SampleTime=.01
  Out1 : Outport  Orientation=down
  wires:
  Relational Operator2/1 -> Switch3/2
  In1/1 -> Switch3/1, Relational Operator2/1, Relational Operator2/2
  Switch3/1 -> Integer Delay3/1, Out1/1
  Integer Delay3/1 -> Switch3/3

== system controlMCUSlugsMKII/Inner Loop/ Navigation/Navigation/Compute Lateral Error/Subsystem3/Protect NaNs ==
  In1 : Inport
  Integer Delay3 : simulink/Discrete/Integer Delay  Orientation=left  vinit=0.0  samptime=T  NumDelays=1
  Relational Operator2 : RelationalOperator  Operator===  LogicOutDataTypeMode=Specify via dialog
  Switch3 : Switch  Criteria=u2 > Threshold  Threshold=0.3  SampleTime=.01
  Out1 : Outport  Orientation=down
  wires:
  Relational Operator2/1 -> Switch3/2
  In1/1 -> Switch3/1, Relational Operator2/1, Relational Operator2/2
  Switch3/1 -> Integer Delay3/1, Out1/1
  Integer Delay3/1 -> Switch3/3

== system controlMCUSlugsMKII/Inner Loop/ Navigation/Navigation/Compute WP Index/Compute P/Compute R ==
  U_com : Inport
  Product : Product  OutDataTypeMode=single  RndMeth=Zero
  Product1 : Product  Inputs=*/  OutDataTypeMode=single  RndMeth=Zero
  gravity1 : Constant  Value=ISA_g*tan(bankCommandLimit)  OutDataTypeMode=single
  R : Outport
  wires:
  Product1/1 -> R/1
  U_com/1 -> Product/2, Product/1
  gravity1/1 -> Product1/2
  Product/1 -> Product1/1

== system controlMCUSlugsMKII/Inner Loop/ Navigation/Navigation/Compute WP Index/Compute P/Compute T  in Frenet ==
  Pos 1 : Inport
  Pos 2 : Inport  Port=2
  Add : Sum  Inputs=-+  OutScaling=2^-10
  Normalize Vector : Subsystem  AncestorBlock=SLUGS_Library/Navigation/Normalize Vector
  T : Outport
  wires:
  Pos 1/1 -> Add/1
  Pos 2/1 -> Add/2
  Add/1 -> Normalize Vector/1(Vector)
  Normalize Vector/1(Normalized) -> T/1

== system controlMCUSlugsMKII/Inner Loop/ Navigation/Navigation/Compute WP Index/Compute P/Geod2LTP1 ==
  GS Lat,Lon : Inport
  GS ECEF : Inport  Port=2
  "Lat, deg(GPS)" : Inport  Port=3
  "Lon, deg(GPS)" : Inport  Port=4
  Hight,m(GPS) : Inport  Port=5
  ECEF2LTP (UEN) : Subsystem
      mask Display: plot(0,0,100,100,[45,40,35,40,40],[85,95,85,95,40],[85,95,85,95,40],[35,40,45,40,40],[60,40,10,20,10,14],[70,40,10,13,10,20],[56,45],[70,70],[60,60],[50,60],[60,60],[30,40],[50,60],[20,20],[30,40],[20,20],[45,55],[35,25],[75,65],[35,25])
  Geod2ECEF1 : Subsystem  mask{Re=6378137, Rp=6356752.3142}
      mask prompts: Re "Enter equatorial radius, m"; Rp "Enter polar radius,m"
  Mux : Mux  Inputs=3
  Reshape : Reshape  OutputDimensionality=Column vector (2-D)
  Reshape1 : Reshape
  Sum1 : Sum  Inputs=|+-  OutDataTypeMode=single  SaturateOnIntegerOverflow=on
  UEN 2 NEU : Gain  Gain=[0 0 1;0 1 0;1 0 0]  Multiplication=Matrix(K*u)  OutDataTypeMode=Specify via dialog  OutDataType=float('single')  SaturateOnIntegerOverflow=on
  "NEU, m" : Outport
  wires:
  UEN 2 NEU/1 -> Reshape1/1
  Geod2ECEF1/3("Ze, m ") -> Mux/3
  Geod2ECEF1/1("Xe, m ") -> Mux/1
  Geod2ECEF1/2("Ye, m ") -> Mux/2
  "Lat, deg(GPS)"/1 -> Geod2ECEF1/2("lat, deg")
  "Lon, deg(GPS)"/1 -> Geod2ECEF1/3(lon,deg)
  GS Lat,Lon/1 -> ECEF2LTP (UEN)/2("Long, Lat")
  GS ECEF/1 -> Sum1/2
  ECEF2LTP (UEN)/1(Out) -> Reshape/1  "Moving Side"
  Hight,m(GPS)/1 -> Geod2ECEF1/1("height, m")
  Mux/1 -> Sum1/1  "r_mov"
  Sum1/1 -> ECEF2LTP (UEN)/1(ECEF coordinates)
  Reshape/1 -> UEN 2 NEU/1
  Reshape1/1 -> "NEU, m"/1

== system controlMCUSlugsMKII/Inner Loop/ Navigation/Navigation/Compute WP Index/Compute P/Get Circles ==
  T1 : Inport
  T2 : Inport  Port=2
  "Wp_to " : Inport  Port=3
  R : Inport  Port=4
  Compute  Circles : Stateflow chart
  Compute CCW Angle From 2 Vectors : Subsystem
  Compute delta Left Turn : Subsystem
  Constant5 : Constant  Value=pi  OutDataTypeMode=single
  Larger than 180? : RelationalOperator  LogicOutDataTypeMode=Boolean  LogicDataType=double()
  Logical Operator : Logic  Operator=NOT  AllPortsSameDT=off  OutDataTypeMode=Boolean
  Merge4 : Merge
  Subsystem5 : SLUGS_Library/Subsystem5  SystemSampleTime=-1
  To Workspace : ToWorkspace  VariableName=O  SampleTime=-1  SaveFormat=Structure
  To Workspace1 : ToWorkspace  VariableName=P  SampleTime=-1  SaveFormat=Structure
  To Workspace2 : ToWorkspace  VariableName=Pch  SampleTime=-1  SaveFormat=Structure
  To Workspace3 : ToWorkspace  VariableName=PchB  SampleTime=-1  SaveFormat=Structure
  compute delta Right Turn : Subsystem
  P : Outport
  wires:
  Subsystem5/2 -> Compute  Circles/2(cd)
  Subsystem5/1 -> Compute  Circles/1(sd)
  Logical Operator/1 -> Compute delta Left Turn/Enable
  Larger than 180?/1 -> Logical Operator/1, compute delta Right Turn/Enable
  Constant5/1 -> Larger than 180?/2
  Compute  Circles/4(PchB) -> To Workspace3/1
  Compute  Circles/3(Pch) -> To Workspace2/1
  Compute  Circles/2(P) -> To Workspace1/1, P/1
  Compute  Circles/1(O) -> To Workspace/1
  "Wp_to "/1 -> Compute  Circles/3(WP1)
  R/1 -> Compute  Circles/4(R)
  Compute delta Left Turn/1(delta) -> Merge4/2
  compute delta Right Turn/1(delta) -> Merge4/1
  Merge4/1 -> Subsystem5/1
  T2/1 -> Compute CCW Angle From 2 Vectors/2(V), Compute  Circles/6(T2)
  Compute CCW Angle From 2 Vectors/1(CCW Ang) -> Larger than 180?/1, compute delta Right Turn/1(gamma), Compute delta Left Turn/1(gamma)  "gamma"
  T1/1 -> Compute CCW Angle From 2 Vectors/1(U), Compute  Circles/5(T1)

== system controlMCUSlugsMKII/Inner Loop/ Navigation/Navigation/Compute WP Index/Compute P/get WP Coord from Index ==
  WP Idx : Inport
  C Function Call : dsPICdrivers/OTHERS/C Function Call  Tag=dsPIC_dsPIC_CFunctionCall  fctName='getWP'  INPUT_SIZE=1  INPUT1=uint8  INPUT2=--  INPUT3=--  OUTPUT_SIZE=3  OUTPUT1=real32  SampleTime=-1  InputType=[ 2 ]  OutputType=[ 7 ]  FctDeclaration=extern void getWP(uint8_T u1,real32_T* y1);  FctCall=getWP(%u1, *%y1);  OrderingInOutPopup=None
  WP Coord : Outport
  wires:
  C Function Call/1 -> WP Coord/1
  WP Idx/1 -> C Function Call/1

== system controlMCUSlugsMKII/Inner Loop/ Navigation/Navigation/Compute WP Index/Grab IC/Compute GS Location ==
  GS Location : Inport
  Demux : Demux  Outputs=3
  Geod2ECEF1 : Subsystem  mask{Re=6378137, Rp=6356752.3142}
      mask prompts: Re "Enter equatorial radius, m"; Rp "Enter polar radius,m"
  Mux1 : Mux  Inputs=2
  Mux2 : Mux  Inputs=3
  "Lat, Lon" : Outport
  R_in : Outport  Port=2
  wires:
  Mux2/1 -> R_in/1  "R_in"
  Mux1/1 -> "Lat, Lon"/1
  GS Location/1 -> Demux/1
  Demux/3 -> Geod2ECEF1/3(lon,deg), Mux1/1
  Demux/2 -> Geod2ECEF1/2("lat, deg"), Mux1/2
  Demux/1 -> Geod2ECEF1/1("height, m")
  Geod2ECEF1/2("Ye, m ") -> Mux2/2
  Geod2ECEF1/1("Xe, m ") -> Mux2/1
  Geod2ECEF1/3("Ze, m ") -> Mux2/3

== system controlMCUSlugsMKII/Inner Loop/ Navigation/Navigation/Compute WP Index/Grab IC/get GS Location (WP 11 is GS) ==
  WP Idx : Inport
  C Function Call : dsPICdrivers/OTHERS/C Function Call  Tag=dsPIC_dsPIC_CFunctionCall  fctName='getWP'  INPUT_SIZE=1  INPUT1=uint8  INPUT2=--  INPUT3=--  OUTPUT_SIZE=3  OUTPUT1=real32  SampleTime=-1  InputType=[ 2 ]  OutputType=[ 7 ]  FctDeclaration=extern void getWP(uint8_T u1,real32_T* y1);  FctCall=getWP(%u1, *%y1);  OrderingInOutPopup=None
  WP Coord : Outport
  wires:
  WP Idx/1 -> C Function Call/1
  C Function Call/1 -> WP Coord/1

== system controlMCUSlugsMKII/Inner Loop/ Navigation/Navigation/Compute WP Index/Switch when  in Line Segment/Compute  Projection ==
  Puav : Inport
  WP0 : Inport  Port=2
  T : Inport  Port=3
  Protect NaNs : Subsystem
  Subsystem3 : Subsystem  AncestorBlock=SLUGS_Library/Subsystem3
  Subtract : Sum  Inputs=+-  OutDataTypeMode=single  OutScaling=2^-10
  Dg : Outport
  wires:
  Subsystem3/1(x dot y) -> Protect NaNs/1(In1)
  T/1 -> Subsystem3/2(y)
  Subtract/1 -> Subsystem3/1(x)
  WP0/1 -> Subtract/2
  Puav/1 -> Subtract/1
  Protect NaNs/1(Out1) -> Dg/1

== system controlMCUSlugsMKII/Inner Loop/ Navigation/Navigation/Compute WP Index/Switch when  in Line Segment/Compute Total Run ==
  WP1 : Inport
  "WP0  " : Inport  Port=2
  P : Inport  Port=3
  Enable : EnablePort
  Compute Distance : Subsystem  AncestorBlock=SLUGS_Library/Navigation/Compute Distance
  Protect NaNs : Subsystem
  Subtract1 : Sum  Inputs=-+  OutDataTypeMode=single  OutScaling=2^-10
  Tot Run : Outport  InitialOutput=150
  wires:
  Subtract1/1 -> Protect NaNs/1(In1)
  P/1 -> Subtract1/1
  Compute Distance/1(Dist) -> Subtract1/2
  "WP0  "/1 -> Compute Distance/1(Pos 1)
  WP1/1 -> Compute Distance/2(Pos 2)
  Protect NaNs/1(Out1) -> Tot Run/1

== system controlMCUSlugsMKII/Inner Loop/ Navigation/Navigation/Compute WP Index/Switch when  in Line Segment/Subsystem1 ==
  swInc : Inport  Orientation=down
  Add : Sum  Orientation=left  Inputs=3  OutScaling=2^-10
  IC : InitialCondition  Orientation=down
  Integer Delay1 : simulink/Discrete/Integer Delay  Orientation=left  vinit=1  samptime=-1  NumDelays=1
  Integer Delay2 : simulink/Discrete/Integer Delay  Orientation=left  vinit=1  samptime=-1  NumDelays=2
  swEna : Outport  Orientation=left
  wires:
  Integer Delay1/1 -> Add/1
  Integer Delay2/1 -> Add/2
  IC/1 -> Integer Delay1/1, Add/3, Integer Delay2/1
  Add/1 -> swEna/1
  swInc/1 -> IC/1

== system controlMCUSlugsMKII/Inner Loop/ Navigation/Navigation/Compute WP Index/Switch when  in Line Segment/WP Update ==
  XYZ : Inport
  Demux : Demux  Outputs=3
  Detect Change : Subsystem
  Detect Change1 : Subsystem
  Detect Change2 : Subsystem
  Saturation1 : Saturate  UpperLimit=1  LowerLimit=0  SampleTime=T
  Sum : Sum  Inputs=3
  Update? : Outport
  wires:
  Saturation1/1 -> Update?/1
  XYZ/1 -> Demux/1
  Sum/1 -> Saturation1/1
  Detect Change2/1(change?) -> Sum/3
  Detect Change1/1(change?) -> Sum/2
  Detect Change/1(change?) -> Sum/1
  Demux/3 -> Detect Change2/1(Data)
  Demux/2 -> Detect Change1/1(Data)
  Demux/1 -> Detect Change/1(Data)

== system controlMCUSlugsMKII/Inner Loop/ Navigation/Navigation/Get Wps Compute Frenet/Geod2LTP1/ECEF2LTP (UEN) ==
  ECEF coordinates : Inport
  "Long, Lat" : Inport  Port=2
  Deg2R : Gain  Gain=pi/180  SaturateOnIntegerOverflow=on
  Demux3 : Demux  Outputs=2
  From Body to Universal1 : Subsystem
  Product1 : Product  Multiplication=Matrix(*)  SaturateOnIntegerOverflow=on  InputSameDT=on
  Out : Outport
  wires:
  "Long, Lat"/1 -> Deg2R/1
  Product1/1 -> Out/1
  Demux3/2 -> From Body to Universal1/2(lat)
  Demux3/1 -> From Body to Universal1/1(long)
  Deg2R/1 -> Demux3/1
  ECEF coordinates/1 -> Product1/2
  From Body to Universal1/1(DCM) -> Product1/1

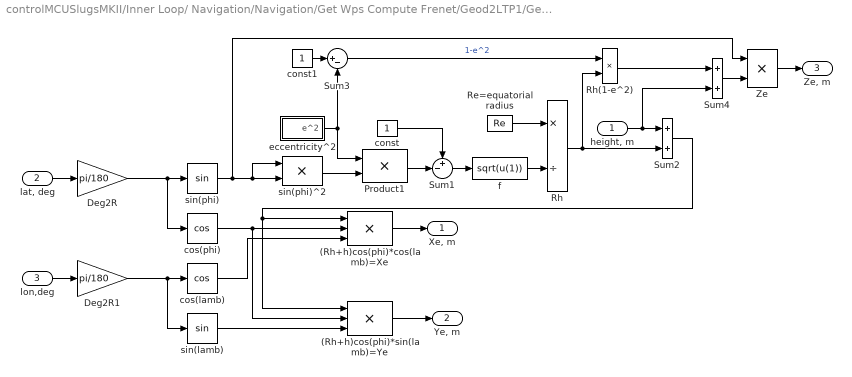
== system controlMCUSlugsMKII/Inner Loop/ Navigation/Navigation/Get Wps Compute Frenet/Geod2LTP1/Geod2ECEF1 ==
  "height, m" : Inport
  "lat, deg" : Inport  Port=2
  lon,deg : Inport  Port=3
  (Rh+h)cos(phi)*cos(lamb)=Xe : Product  Inputs=3  OutDataTypeMode=single  SaturateOnIntegerOverflow=on  InputSameDT=on
  (Rh+h)cos(phi)*sin(lamb)=Ye : Product  Inputs=3  OutDataTypeMode=single  SaturateOnIntegerOverflow=on  InputSameDT=on
  Deg2R : Gain  Gain=pi/180  OutDataTypeMode=Specify via dialog  OutDataType=float('single')  SaturateOnIntegerOverflow=on
  Deg2R1 : Gain  Gain=pi/180  OutDataTypeMode=Specify via dialog  OutDataType=float('single')  SaturateOnIntegerOverflow=on
  Product1 : Product  SaturateOnIntegerOverflow=on  InputSameDT=on
  Re=equatorial radius : Constant  Value=Re  OutDataTypeMode=single
  Rh : Product  Inputs=*/  OutDataTypeMode=single  SaturateOnIntegerOverflow=on  InputSameDT=on
  Rh(1-e^2) : Product  OutDataTypeMode=single  SaturateOnIntegerOverflow=on  InputSameDT=on
  Sum1 : Sum  Inputs=+-|  SaturateOnIntegerOverflow=on  InputSameDT=on
  Sum2 : Sum  SaturateOnIntegerOverflow=on  InputSameDT=on
      settings: AttributesFormatString=Rh+h
  Sum3 : Sum  Inputs=|+-  SaturateOnIntegerOverflow=on  InputSameDT=on
  Sum4 : Sum  OutDataTypeMode=single  SaturateOnIntegerOverflow=on  InputSameDT=on
      settings: AttributesFormatString=(1-e^2)Rh+h
  Ze : Product  OutDataTypeMode=single  SaturateOnIntegerOverflow=on  InputSameDT=on
  const : Constant  OutDataTypeMode=single
  const1 : Constant  OutDataTypeMode=single
  cos(lamb) : Trigonometry  Operator=cos
  cos(phi) : Trigonometry  Operator=cos
  eccentricity^2 : Subsystem
  f : Fcn  Expr=sqrt(u(1))
  sin(lamb) : Trigonometry
  sin(phi) : Trigonometry
  sin(phi)^2 : Product  SaturateOnIntegerOverflow=on  InputSameDT=on
  "Xe, m " : Outport
  "Ye, m " : Outport  Port=2
  "Ze, m " : Outport  Port=3
  wires:
  "lat, deg"/1 -> Deg2R/1
  sin(phi)/1 -> sin(phi)^2/1, sin(phi)^2/2, Ze/1
  f/1 -> Rh/2
  Re=equatorial radius/1 -> Rh/1
  Rh/1 -> Sum2/2, Rh(1-e^2)/2
  Product1/1 -> Sum1/2
  Sum1/1 -> f/1
  const/1 -> Sum1/1
  "height, m"/1 -> Sum4/2, Sum2/1
  eccentricity^2/1(e^2) -> Product1/1, Sum3/2
  sin(phi)^2/1 -> Product1/2
  const1/1 -> Sum3/1
  Sum3/1 -> Rh(1-e^2)/1  "1-e^2"
  Rh(1-e^2)/1 -> Sum4/1
  Sum4/1 -> Ze/2
  lon,deg/1 -> Deg2R1/1
  cos(phi)/1 -> (Rh+h)cos(phi)*cos(lamb)=Xe/2, (Rh+h)cos(phi)*sin(lamb)=Ye/2
  cos(lamb)/1 -> (Rh+h)cos(phi)*cos(lamb)=Xe/3
  sin(lamb)/1 -> (Rh+h)cos(phi)*sin(lamb)=Ye/3
  Ze/1 -> "Ze, m "/1
  Deg2R/1 -> cos(phi)/1, sin(phi)/1
  Deg2R1/1 -> cos(lamb)/1, sin(lamb)/1
  Sum2/1 -> (Rh+h)cos(phi)*sin(lamb)=Ye/1, (Rh+h)cos(phi)*cos(lamb)=Xe/1
  (Rh+h)cos(phi)*cos(lamb)=Xe/1 -> "Xe, m "/1
  (Rh+h)cos(phi)*sin(lamb)=Ye/1 -> "Ye, m "/1

== system controlMCUSlugsMKII/Inner Loop/ Navigation/Navigation/Get Wps Compute Frenet/Geod2LTP2/ECEF2LTP (UEN) ==
  ECEF coordinates : Inport
  "Long, Lat" : Inport  Port=2
  Deg2R : Gain  Gain=pi/180  SaturateOnIntegerOverflow=on
  Demux3 : Demux  Outputs=2
  From Body to Universal1 : Subsystem
  Product1 : Product  Multiplication=Matrix(*)  SaturateOnIntegerOverflow=on  InputSameDT=on
  Out : Outport
  wires:
  "Long, Lat"/1 -> Deg2R/1
  Product1/1 -> Out/1
  Demux3/2 -> From Body to Universal1/2(lat)
  Demux3/1 -> From Body to Universal1/1(long)
  Deg2R/1 -> Demux3/1
  ECEF coordinates/1 -> Product1/2
  From Body to Universal1/1(DCM) -> Product1/1

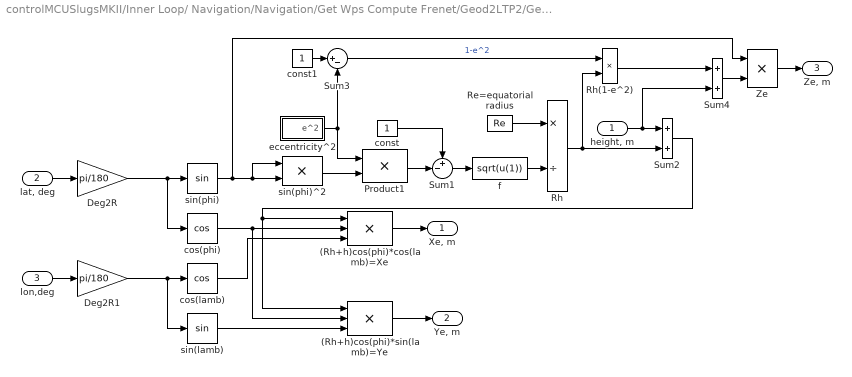
== system controlMCUSlugsMKII/Inner Loop/ Navigation/Navigation/Get Wps Compute Frenet/Geod2LTP2/Geod2ECEF1 ==
  "height, m" : Inport
  "lat, deg" : Inport  Port=2
  lon,deg : Inport  Port=3
  (Rh+h)cos(phi)*cos(lamb)=Xe : Product  Inputs=3  OutDataTypeMode=single  SaturateOnIntegerOverflow=on  InputSameDT=on
  (Rh+h)cos(phi)*sin(lamb)=Ye : Product  Inputs=3  OutDataTypeMode=single  SaturateOnIntegerOverflow=on  InputSameDT=on
  Deg2R : Gain  Gain=pi/180  OutDataTypeMode=Specify via dialog  OutDataType=float('single')  SaturateOnIntegerOverflow=on
  Deg2R1 : Gain  Gain=pi/180  OutDataTypeMode=Specify via dialog  OutDataType=float('single')  SaturateOnIntegerOverflow=on
  Product1 : Product  SaturateOnIntegerOverflow=on  InputSameDT=on
  Re=equatorial radius : Constant  Value=Re  OutDataTypeMode=single
  Rh : Product  Inputs=*/  OutDataTypeMode=single  SaturateOnIntegerOverflow=on  InputSameDT=on
  Rh(1-e^2) : Product  OutDataTypeMode=single  SaturateOnIntegerOverflow=on  InputSameDT=on
  Sum1 : Sum  Inputs=+-|  SaturateOnIntegerOverflow=on  InputSameDT=on
  Sum2 : Sum  SaturateOnIntegerOverflow=on  InputSameDT=on
      settings: AttributesFormatString=Rh+h
  Sum3 : Sum  Inputs=|+-  SaturateOnIntegerOverflow=on  InputSameDT=on
  Sum4 : Sum  OutDataTypeMode=single  SaturateOnIntegerOverflow=on  InputSameDT=on
      settings: AttributesFormatString=(1-e^2)Rh+h
  Ze : Product  OutDataTypeMode=single  SaturateOnIntegerOverflow=on  InputSameDT=on
  const : Constant  OutDataTypeMode=single
  const1 : Constant  OutDataTypeMode=single
  cos(lamb) : Trigonometry  Operator=cos
  cos(phi) : Trigonometry  Operator=cos
  eccentricity^2 : Subsystem
  f : Fcn  Expr=sqrt(u(1))
  sin(lamb) : Trigonometry
  sin(phi) : Trigonometry
  sin(phi)^2 : Product  SaturateOnIntegerOverflow=on  InputSameDT=on
  "Xe, m " : Outport
  "Ye, m " : Outport  Port=2
  "Ze, m " : Outport  Port=3
  wires:
  "lat, deg"/1 -> Deg2R/1
  sin(phi)/1 -> sin(phi)^2/1, sin(phi)^2/2, Ze/1
  f/1 -> Rh/2
  Re=equatorial radius/1 -> Rh/1
  Rh/1 -> Sum2/2, Rh(1-e^2)/2
  Product1/1 -> Sum1/2
  Sum1/1 -> f/1
  const/1 -> Sum1/1
  "height, m"/1 -> Sum4/2, Sum2/1
  eccentricity^2/1(e^2) -> Product1/1, Sum3/2
  sin(phi)^2/1 -> Product1/2
  const1/1 -> Sum3/1
  Sum3/1 -> Rh(1-e^2)/1  "1-e^2"
  Rh(1-e^2)/1 -> Sum4/1
  Sum4/1 -> Ze/2
  lon,deg/1 -> Deg2R1/1
  cos(phi)/1 -> (Rh+h)cos(phi)*cos(lamb)=Xe/2, (Rh+h)cos(phi)*sin(lamb)=Ye/2
  cos(lamb)/1 -> (Rh+h)cos(phi)*cos(lamb)=Xe/3
  sin(lamb)/1 -> (Rh+h)cos(phi)*sin(lamb)=Ye/3
  Ze/1 -> "Ze, m "/1
  Deg2R/1 -> cos(phi)/1, sin(phi)/1
  Deg2R1/1 -> cos(lamb)/1, sin(lamb)/1
  Sum2/1 -> (Rh+h)cos(phi)*sin(lamb)=Ye/1, (Rh+h)cos(phi)*cos(lamb)=Xe/1
  (Rh+h)cos(phi)*cos(lamb)=Xe/1 -> "Xe, m "/1
  (Rh+h)cos(phi)*sin(lamb)=Ye/1 -> "Ye, m "/1

== system controlMCUSlugsMKII/Inner Loop/ Navigation/Navigation/Park, Deyst & How Lat Accel Cmd/Compute Eta/Subsystem6 ==
  x : Inport
  C Function Call : dsPICdrivers/OTHERS/C Function Call  Tag=dsPIC_dsPIC_CFunctionCall  fctName='myAsin'  INPUT_SIZE=1  INPUT1=real32  INPUT2=--  INPUT3=--  OUTPUT_SIZE=1  OUTPUT1=real32  SampleTime=-1  InputType=[ 7 ]  OutputType=[ 7 ]  FctDeclaration=extern real32_T myAsin(real32_T u1);  FctCall=%y1 = myAsin(%u1);  OrderingInOutPopup=None
  Environment Controller : simulink/Signal Routing/Environment Controller  SystemSampleTime=-1
  Protect NaNs : Subsystem
  Trigonometric Function : Trigonometry  Operator=asin
  "[-1,1]" : Saturate  UpperLimit=0.9999  LowerLimit=-0.999
  asin(x) : Outport
  wires:
  "[-1,1]"/1 -> C Function Call/1, Trigonometric Function/1
  x/1 -> Protect NaNs/1(In1)
  Trigonometric Function/1 -> Environment Controller/1
  C Function Call/1 -> Environment Controller/2
  Environment Controller/1 -> asin(x)/1
  Protect NaNs/1(Out1) -> "[-1,1]"/1
